simulink library "NEXTCAR_Library"  (R2017a)
settings: Solver=VariableStepAuto  StartTime=0.0  StopTime=10.0  RelTol=1e-3
settings Model: Creator=joreADM  LastModifiedBy=joreADM

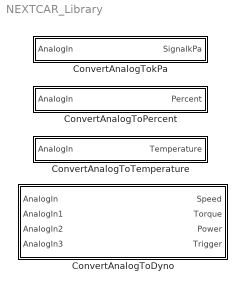
== system NEXTCAR_Library ==
  ConvertAnalogToDyno : Subsystem  mask(Voltage [V] to Dyno Parameter Conversion){speed_max=0, torque_max=0, power_max=0, trigger_max=0}
      mask prompts: speed_max "Maximum Speed [RPM]"; torque_max "Maximum Torque [ft-lbf]"; power_max "Maximum Power [HP]"; trigger_max "Maximum Trigger [int]"
      mask help: Converts the input analog voltages [V] to corresponding Dyno measurements. Specify the maximum value for each measurement in the dialog fields below.
      mask Display:
      | color('white');
      | dispStr1 = strcat(strcat('Vmax=',get_param(gcb,'speed_max')),'[RPM]');
      | dispStr2 = strcat(strcat('Tqmax=',get_param(gcb,'torque_max')),'[ft-lbf]');
      | dispStr3 = strcat(strcat('Pmax=',get_param(gcb,'power_max')),'[HP]');
      | dispStr4 = strcat(strcat('Trmax=',get_param(gcb,'trigger_max')),'[int]');
      | dispStr = strvcat(' ',dispStr1,dispStr2,dispStr3,dispStr4);
      | disp(dispStr);
      | port_label('input',1,'Analog_[V]');
      | port_label('input',2,'Analog_[V]');
      | port_label('input',3,'Analog_[V]');
      | port_label('input',4,'Analog_[V]');
      | port_label('output',1,'Speed [RPM]');
      | port_label('output',2,'Torque [ft-lbf]');
      | port_label('output',3,'Power [HP]');
      | port_label('output',4,'Trigger [int]');
  ConvertAnalogToPercent : Subsystem  mask(Voltage [V] to Percentage [%] Conversion){V_Max=0}
      mask prompts: V_Max "Voltage Range [V]"
      mask help: Specify the maximum voltage value in [V] to convert from an input analog value to a corresponding percentage value output in [%].
      mask Display:
      | color('white');
      | dispStr = strcat(strcat('Vmax=',get_param(gcb,'V_Max')),'[V]');
      | disp(dispStr);
      | port_label('input',1,'Analog_[V]');
      | port_label('output',1,'[%]');
  ConvertAnalogToTemperature : Subsystem  mask(Voltage [V] to Temperature [C] Conversion){}
      mask help: Converts the input analog voltage [V] to the corresponding temperature value in [C].
      mask Display:
      | color('white');
      | port_label('input',1,'Analog_[V]');
      | port_label('output',1,'Temperature [C]');
  ConvertAnalogTokPa : Subsystem  mask(Voltage [V] to Pressure [kPa] Conversion){P_Max=0}
      mask prompts: P_Max "Pressure Range [bar]"
      mask help: Specify the maximum pressure value in [bar] below to convert from an analog voltage input to the corresponding pressure value in [kPa].
      mask Display:
      | color('white');
      | dispStr = strcat(strcat('Pmax=',get_param(gcb,'P_Max')),'[bar]');
      | disp(dispStr);
      | port_label('input',1,'Analog_[V]');
      | port_label('output',1,'P_[kPa]');

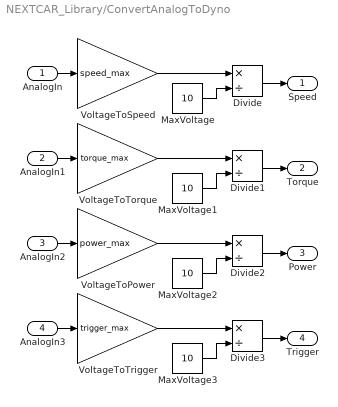
== system NEXTCAR_Library/ConvertAnalogToDyno ==
  AnalogIn : Inport
  AnalogIn1 : Inport  Port=2
  AnalogIn2 : Inport  Port=3
  AnalogIn3 : Inport  Port=4
  Divide{,1..3} (4 alike) : Product  Inputs=*/
  MaxVoltage{,1..3} (4 alike) : Constant  Value=10
  VoltageToPower : Gain  Gain=power_max
  VoltageToSpeed : Gain  Gain=speed_max
  VoltageToTorque : Gain  Gain=torque_max
  VoltageToTrigger : Gain  Gain=trigger_max
  Speed : Outport
  Torque : Outport  Port=2
  Power : Outport  Port=3
  Trigger : Outport  Port=4
  wires:
  AnalogIn/1 -> VoltageToSpeed/1
  AnalogIn1/1 -> VoltageToTorque/1
  AnalogIn2/1 -> VoltageToPower/1
  AnalogIn3/1 -> VoltageToTrigger/1
  VoltageToSpeed/1 -> Divide/1
  Divide/1 -> Speed/1
  MaxVoltage/1 -> Divide/2
  VoltageToTorque/1 -> Divide1/1
  MaxVoltage1/1 -> Divide1/2
  Divide1/1 -> Torque/1
  Divide2/1 -> Power/1
  MaxVoltage2/1 -> Divide2/2
  VoltageToPower/1 -> Divide2/1
  VoltageToTrigger/1 -> Divide3/1
  MaxVoltage3/1 -> Divide3/2
  Divide3/1 -> Trigger/1

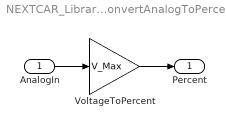
== system NEXTCAR_Library/ConvertAnalogToPercent ==
  AnalogIn : Inport
  VoltageToPercent : Gain  Gain=V_Max
  Percent : Outport
  wires:
  AnalogIn/1 -> VoltageToPercent/1
  VoltageToPercent/1 -> Percent/1

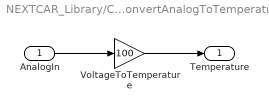
== system NEXTCAR_Library/ConvertAnalogToTemperature ==
  AnalogIn : Inport
  VoltageToTemperature : Gain  Gain=100
  Temperature : Outport
  wires:
  VoltageToTemperature/1 -> Temperature/1
  AnalogIn/1 -> VoltageToTemperature/1

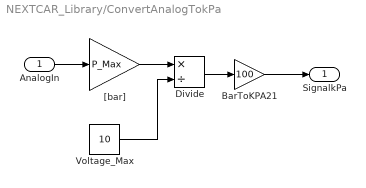
== system NEXTCAR_Library/ConvertAnalogTokPa ==
  AnalogIn : Inport
  BarToKPA21 : Gain  Gain=100
  Divide : Product  Inputs=*/
  Voltage_Max : Constant  Value=10
  "[bar]" : Gain  Gain=P_Max
  SignalkPa : Outport
  wires:
  Voltage_Max/1 -> Divide/2
  "[bar]"/1 -> Divide/1
  AnalogIn/1 -> "[bar]"/1
  BarToKPA21/1 -> SignalkPa/1
  Divide/1 -> BarToKPA21/1
